simulink model "VCU2BMS"  (R2019b)
settings: Solver=VariableStepAuto  StartTime=0.0  StopTime=10.0  RelTol=1e-3
undefined symbols (not defined in the file or in its folder): sigbuilder_block
libraries: simulink x1
settings Model: Creator=YJR  LastModifiedBy=YJR

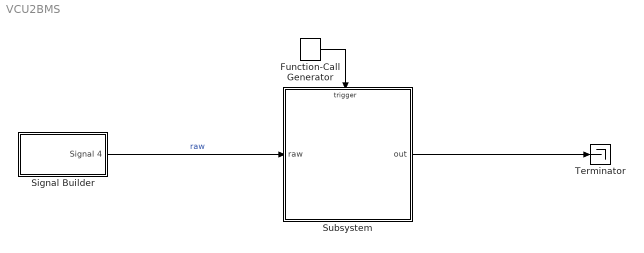
== system VCU2BMS ==
  Function-Call Generator : simulink/Ports & Subsystems/Function-Call Generator  sample_time=0.01  numberOfIterations=1
  Signal Builder : Subsystem  Tag=STV Subsys  LoadFcn=sigbuilder_block('load');  StartFcn=sigbuilder_block('start');  StopFcn=sigbuilder_block('stop');  ClipboardFcn=sigbuilder_block('clipboard');  mask(Sigbuilder block){tuvar=[0:10]}
      mask help: Simulink:masks:SigbuilderBlock_MD
      mask init:
      | if ~strcmp(get_param(bdroot(gcbh),'SimulationStatus'),'stopped') tuvar = sigbuilder_block('maskInit'); end
      settings: CopyFcn=sigbuilder_block('copy');  DeleteFcn=sigbuilder_block('delete');  ModelCloseFcn=sigbuilder_block('modelClose');  PreSaveFcn=sigbuilder_block('preSave');  PauseFcn=sigbuilder_block('pause');  ContinueFcn=sigbuilder_block('continue');  NameChangeFcn=sigbuilder_block('namechange');  OpenFcn=sigbuilder_block('open',[437.6 199.2 550.4 400 ]);  CloseFcn=sigbuilder_block('close');
      mask Display: plot(0, 0, 100, 100,[2, 2, 32, 32, 2], [68, 8, 8, 68, 68],[32, 2], [38, 38], [32, 19, 2],[53, 60, 44], [32, 17, 17, 2],[16, 16, 31, 31]);txt = getActiveGroup(gcbh);text(2, 100, txt,'verticalAlignment', 'top');
  Subsystem : Subsystem
  Terminator : Terminator
  wires:
  Signal Builder/1(Signal 4) -> Subsystem/1(raw)  "raw"
  Subsystem/1(out) -> Terminator/1
  Function-Call Generator/1 -> Subsystem/Trigger

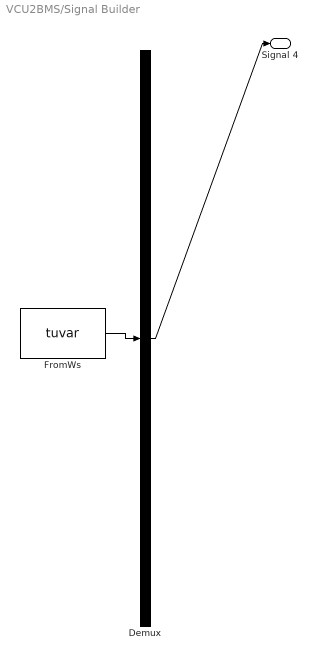
== system VCU2BMS/Signal Builder ==
  Demux : Demux  Tag=STV Demux  Outputs=1
  FromWs : FromWorkspace  Tag=STV FromWs  VariableName=tuvar  SampleTime=0
      SigBuilderData=|
      | common.afterFinalStr = 'Extrapolate'
      | common.sampleTime = 0
      | dataSet.timeRange = [0 10]
      | dataSet.name = 'Group 1'
      | sbobj.Groups.Name = 'Group 1'
      | sbobj.Groups.Signals.Name = 'Signal 4'
      | sbobj.Groups.Signals.XData = [0 1 2 2 3 3 4 4 5 5 6 7 8 8 9 9 10]
      | sbobj.Groups.Signals.YData = [0 0 0 1 1 0 0 1 1 0 0 0 0 1 1 0 0]
  Signal 4 : Outport  Tag=STV Outport
  wires:
  FromWs/1 -> Demux/1
  Demux/1 -> Signal 4/1

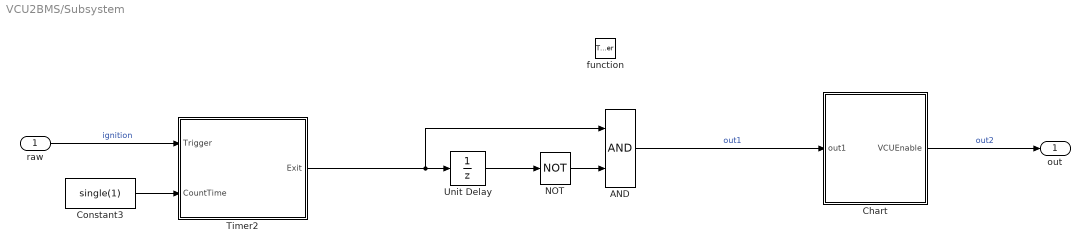
== system VCU2BMS/Subsystem ==
  raw : Inport
  function : TriggerPort  TriggerType=function-call  VariantControl=Variant
  AND : Logic  AllPortsSameDT=off  OutDataTypeStr=boolean
  Chart : Stateflow chart  BlockKeywords=__PRM__SERIALIZED__DATA__:Stateflow Chart,Stateflow Diagram  TreatAsAtomicUnit=on
  Constant3 : Constant  Value=single(1)
  NOT : Logic  Operator=NOT  AllPortsSameDT=off  OutDataTypeStr=boolean
  Timer2 : Stateflow chart  TreatAsAtomicUnit=on
  Unit Delay : UnitDelay  SampleTime=-1  HasFrameUpgradeWarning=on
  out : Outport
  wires:
  Timer2/1(Exit) -> AND/1, Unit Delay/1
  Unit Delay/1 -> NOT/1
  NOT/1 -> AND/2
  AND/1 -> Chart/1(out1)  "out1"
  raw/1 -> Timer2/1(Trigger)  "ignition"
  Constant3/1 -> Timer2/2(CountTime)
  Chart/1(VCUEnable) -> out/1  "out2"

== stateflow chart VCU2BMS/Subsystem/Chart ==
  state STATEON
    state initstate
      en:
      VCUEnable=0;
    state ON
      en:
      VCUEnable=1;
    (default) -> STATEON.initstate
    STATEON.initstate -> ON : after(0.2,sec)[out1]
  state STATEOFF
    state initstate
      en:
      VCUEnable=1;
    state OFF
      en:
      VCUEnable=0;
    (default) -> STATEOFF.initstate
    STATEOFF.initstate -> OFF : after(0.2,sec)[out1]
  (default) -> STATEON
  ON -> STATEOFF
  OFF -> STATEON
  data: out1 input; VCUEnable output

== stateflow chart VCU2BMS/Subsystem/Timer2 ==
  state Trigger
    en:
    x = x + 0.01;
    Exit=0;
  state Out
    en:
    Exit=1;
    x=0;
  state InterState
    en:
    x=0;
  Trigger -> Trigger [order 1] : [Trigger&&x<CountTime]
  Trigger -> Out [order 2] : [x>=CountTime]
  (default) -> Trigger
  Out -> Trigger : [~Trigger]
  InterState -> Trigger : [Trigger]
  Trigger -> InterState [order 3] : [x<CountTime&&~Trigger]
  data: Trigger input; CountTime input; Exit output; x local =0
